simulink model "CoupledTanks"  (Simulink 6.5)
settings: Solver=ode45  StartTime=0.0  StopTime=2000  MaxStep=1e-1  RelTol=1e-3
InitFcn:
  | g = 9.81; %gravitational constant
  | 
  | % showVR = 1; %show VR world
  | % h1_init = 0; %initial condition
  | % h2_init = 0; %initial condition
libraries: vrlib x7
CloseFcn:
  | vrclose all;
  | clear figureVR worldVR;
settings Model: Creator=H  LastModifiedBy=Roubalj

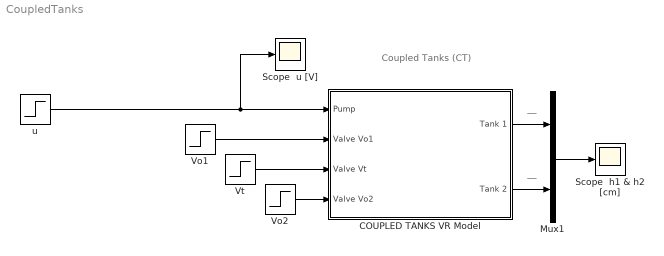
== system CoupledTanks ==
  note: Coupled Tanks (CT)
  note: __
  note: __
  COUPLED TANKS VR Model : Subsystem  mask(Coupled Tanks (CT) in laboratory K26){showVR=on, sfcnParam1=0, sfcnParam2=0}
      mask prompts: showVR "Show VirtualWorld?"; sfcnParam1 "Initial fluid level in the left tank 1   h1(0)  [cm]"; sfcnParam2 "Initial fluid  level in the right tank 2   h2 (0) [cm]"
      mask help:
      | Coupled Tanks (CT) in laboratory K26 - Virtual Reality
      | Real-Time Workshop generated S-function.
      mask Help:
      | Couple Tanks in laboratory K26 - Virtual Reality. <br><br>
      | 
      | 
      | This is a&nbsp;virtual model of the Coupled Tanks apparatus in Laboratory of automatic control
      | theory&nbsp;26 (<a href="http://support.dce.felk.cvut.cz/lab26/" target="_blank">http://support.dce.felk.cvut.cz/lab26/</a>),
      | which consists of a&nbsp;gear-pump, two tanks (left and right), inflow and outflow pipes and transfer (V<sub>t</sub>) and
      | output valves (V<sub>o1</sub>, V<sub>o2</sub>). The&nbsp;left tank is filled with the&nbsp;fluid by the&nbsp;gear-pump
      | controller by the&nbsp;voltage&nbsp;<em>u</em>&nbsp;[V]. The&nbsp;fluid can drain from the&nbsp;left tank through
      | the&nbsp;valve&nbsp;<em>v</em><sub>o1</sub>&nbsp;[%] or can drain to the&nbsp;right tank through the&nbsp;transfer
      | valve&nbsp;<em>v</em><sub>t</sub>&nbsp;[%]. The&nbsp;fluid drains away from the&nbsp;right tank through
      | the&nbsp;valve&nbsp;<em>v</em><sub>o2</sub>&nbsp;[%].<br><br>
      | 
      | The&nbsp;system input are the&nbsp;voltage of the&nbsp;motor of the&nbsp;gear-pump&nbsp;<em>u</em>&nbsp;[V]
      | and the&nbsp;opening of
      | the&nbsp;valves&nbsp;<em>v</em><sub>o1</sub>,&nbsp;<em>v</em><sub>t</sub>,&nbsp;<em>v</em><sub>o2</sub>&nbsp;[%].
      | The&nbsp;system outputs are the&nbsp;levels of the&nbsp;fluid in
      | the&nbsp;tanks&nbsp;<em>h</em><sub>1</sub>,&nbsp;<em>h</em><sub>2</sub>&nbsp;[cm].
      | The&nbsp;dynamics of the&nbsp;gear-pump is neglected. More information can be found on the&nbsp;website
      | <a href="http://support.dce.felk.cvut.cz/lab26/" target="_blank">http://support.dce.felk.cvut.cz/lab26/</a>.<br><br>
      | 
      | 
      | In the mask of the model, it can be set:
      | <ul>
      | <li>Initial fluid level in the left tank</li>
      | <li>Initial fluid level in the right tank.</li>
      | </ul><br><br>
      | 
      | 
      | Copyright: 2008, Jan Kricka, Jirka Roubal, Petr Husek.
      mask CallbackString:
      | if strcmp('off',get_param(gcb,'showVR'))
      |     vrclose all;
      | else
      |     if exist('figureVR')==0
      |         figureVR = vrfigure;
      |     end
      |     if exist('worldVR')==0
      |         worldVR = vrworld('CoupledTanks_VR.WRL');
      |     end
      | 	if isvalid(figureVR)==0
      |         open(worldVR);
      |         figureVR = vrfigure(worldVR,[650 80 550 350]);
      | 	end
      | end||
      mask Display:
      | image(imread('CoupledTanks_Image.jpg'));
      | port_label ('input',1,'u [V]');
      | port_label ('input',2,'Vo1 [-]');
      | port_label ('input',3,'Vt [-]');
      | port_label ('input',4,'Vo2 [-]');
      | port_label ('output',1,'h1 [cm]');
      | port_label ('output',2,'h2 [cm]');
  Mux1 : Mux  Inputs=2
  Scope  h1 & h2 [cm] : Scope
      settings: TimeRange=2000  YMin=0  YMax=30  SaveName=ty  DataFormat=Array  MaxDataPoints=500000
  Scope  u [V] : Scope
      settings: TimeRange=2000  YMin=0  YMax=12  SaveName=tu  DataFormat=Array  MaxDataPoints=500000
  Vo1 : Step  Time=0  After=0  SampleTime=0
  Vo2 : Step  Time=0  After=0.60  SampleTime=0
  Vt : Step  Time=0  SampleTime=0
  u : Step  Time=1000  Before=5  After=5*1.05  SampleTime=0
  wires:
  COUPLED TANKS VR Model/1(Tank 1) -> Mux1/1
  Mux1/1 -> Scope  h1 & h2 [cm]/1
  Vo1/1 -> COUPLED TANKS VR Model/2(Valve Vo1)
  Vt/1 -> COUPLED TANKS VR Model/3(Valve Vt)
  Vo2/1 -> COUPLED TANKS VR Model/4(Valve Vo2)
  u/1 -> Scope  u [V]/1, COUPLED TANKS VR Model/1(Pump)
  COUPLED TANKS VR Model/2(Tank 2) -> Mux1/2

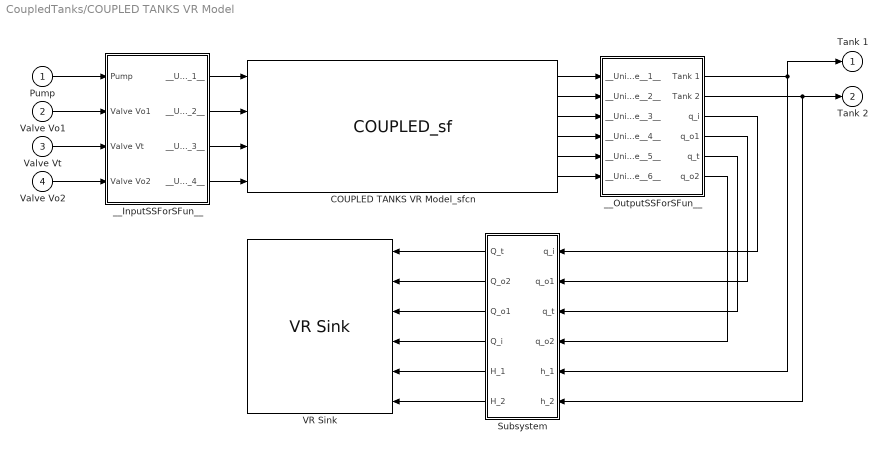
== system CoupledTanks/COUPLED TANKS VR Model ==
  Pump : Inport
  Valve Vo1 : Inport  Port=2
  Valve Vt : Inport  Port=3
  Valve Vo2 : Inport  Port=4
  COUPLED TANKS VR Model_sfcn : S-Function  FunctionName=COUPLED_sf  Parameters=sfcnParam1, sfcnParam2  SFunctionModules=""  mask{rtw_sf_name=COUPLED_sf, showVar=off, sfcnParam1=sfcnParam1, sfcnParam2=sfcnParam2}
      mask prompts: rtw_sf_name "Generated S-function name (model_sf):"; showVar "Show module list"; sfcnParam1 "h1_init:"; sfcnParam2 "h2_init:"
      mask help: Real-Time Workshop generated S-function.
      mask init:
      | displist = '';
      | if ~strcmp(get_param(gcb, 'FunctionName'), rtw_sf_name);
      |   set_param(gcb, 'FunctionName', rtw_sf_name);
      | end
      | % Check if we are generating RTW code
      | rtw_mode = false;
      | if strcmpi(get_param(bdroot(gcb),'SimulationStatus'),'Initializing')
      | 	rtw_mode = strcmpi(get_param(bdroot(gcb),'BuildingRTWCode'),'on') && ...
      | 		~strcmpi(get_param(bdroot(gcb),'TargetStyle'),'SimulationTarget');
      | end
      | if showVar || rtw_mode
      | 	if exist('rtwsfunc') == 2 | exist('rtwsfunc') == 6
      | 		tmplist = rtwsfunc(rtw_sf_name,gcb);
      | 		tmplist = ['\nList of Modules:\n', tmplist];
      | 	elseif showVar
      | 		tmplist = '\nList of Modules:\nRTW not licensed\n';
      |  	end
      | end
      | if showVar
      |   displist = tmplist;
      | end
      settings: CopyFcn=set_param(gcb,'LinkStatus','none');
      mask Help: helpview([docroot,'\toolbox\rtw\helptargets.map'],'rtw_Sfunc_target');
      mask Display:
      | port_label('input',1,'Pump');
      | port_label('input',2,'Valve Vo1');
      | port_label('input',3,'Valve Vt');
      | port_label('input',4,'Valve Vo2');
      | port_label('output',1,'Tank 1');
      | port_label('output',2,'Tank 2');
      | port_label('output',3,'q_i');
      | port_label('output',4,'q_o1');
      | port_label('output',5,'q_t');
      | port_label('output',6,'q_o2');
  Subsystem : Subsystem  Orientation=left
  VR Sink : vrlib/VR Sink  Orientation=left  SampleTime=-1  ViewEnable=on  RemoteChange=off  RemoteView=on  FieldsWritten=Valve_t.rotation.4.1.double#Valve_o2.rotation.4.1.double#Valve_o1.rotation.4.1.double#Pump.rotation.4.1.double#water1.scale.3.1.double#water2.scale.3.1.double  WorldFileName=CoupledTanks_VR.WRL  AutoView=off  FigureProperties={}
  __InputSSForSFun__ : Subsystem
  __OutputSSForSFun__ : Subsystem
  Tank 1 : Outport  PortDimensions=1  SampleTime=[-1 0]  DataType=double
  Tank 2 : Outport  Port=2  PortDimensions=1  SampleTime=[-1 0]  DataType=double
  wires:
  __OutputSSForSFun__/6(q_o2) -> Subsystem/4(q_o2)
  __OutputSSForSFun__/5(q_t) -> Subsystem/3(q_t)
  __OutputSSForSFun__/4(q_o1) -> Subsystem/2(q_o1)
  __OutputSSForSFun__/3(q_i) -> Subsystem/1(q_i)
  Subsystem/2(Q_o2) -> VR Sink/2
  Subsystem/3(Q_o1) -> VR Sink/3
  Subsystem/4(Q_i) -> VR Sink/4
  Subsystem/1(Q_t) -> VR Sink/1
  Subsystem/6(H_2) -> VR Sink/6
  Subsystem/5(H_1) -> VR Sink/5
  __OutputSSForSFun__/2(Tank 2) -> Subsystem/6(h_2), Tank 2/1
  __OutputSSForSFun__/1(Tank 1) -> Tank 1/1, Subsystem/5(h_1)
  COUPLED TANKS VR Model_sfcn/6 -> __OutputSSForSFun__/6(__UniqueInportName__6__)
  COUPLED TANKS VR Model_sfcn/5 -> __OutputSSForSFun__/5(__UniqueInportName__5__)
  COUPLED TANKS VR Model_sfcn/4 -> __OutputSSForSFun__/4(__UniqueInportName__4__)
  COUPLED TANKS VR Model_sfcn/3 -> __OutputSSForSFun__/3(__UniqueInportName__3__)
  COUPLED TANKS VR Model_sfcn/2 -> __OutputSSForSFun__/2(__UniqueInportName__2__)
  COUPLED TANKS VR Model_sfcn/1 -> __OutputSSForSFun__/1(__UniqueInportName__1__)
  __InputSSForSFun__/4(__UniqueOutportName__4__) -> COUPLED TANKS VR Model_sfcn/4
  __InputSSForSFun__/3(__UniqueOutportName__3__) -> COUPLED TANKS VR Model_sfcn/3
  __InputSSForSFun__/2(__UniqueOutportName__2__) -> COUPLED TANKS VR Model_sfcn/2
  __InputSSForSFun__/1(__UniqueOutportName__1__) -> COUPLED TANKS VR Model_sfcn/1
  Valve Vo2/1 -> __InputSSForSFun__/4(Valve Vo2)
  Valve Vt/1 -> __InputSSForSFun__/3(Valve Vt)
  Valve Vo1/1 -> __InputSSForSFun__/2(Valve Vo1)
  Pump/1 -> __InputSSForSFun__/1(Pump)

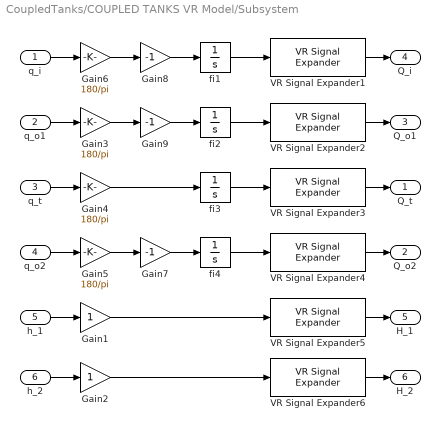
== system CoupledTanks/COUPLED TANKS VR Model/Subsystem ==
  q_i : Inport
  q_o1 : Inport  Port=2
  q_t : Inport  Port=3
  q_o2 : Inport  Port=4
  h_1 : Inport  Port=5
  h_2 : Inport  Port=6
  Gain1 : Gain
  Gain2 : Gain
  Gain{3..6} (4 alike) : Gain  Gain=180/pi
  Gain7 : Gain  Gain=-1
  Gain8 : Gain  Gain=-1
  Gain9 : Gain  Gain=-1
  VR Signal Expander{1..4} (4 alike) : vrlib/VR Signal Expander  SystemSampleTime=-1  outwidth=4  outidx=[4]
  VR Signal Expander5 : vrlib/VR Signal Expander  SystemSampleTime=-1  outwidth=3  outidx=[2]
  VR Signal Expander6 : vrlib/VR Signal Expander  SystemSampleTime=-1  outwidth=3  outidx=[2]
  fi{1..4} (4 alike) : Integrator
  Q_t : Outport
  Q_o2 : Outport  Port=2
  Q_o1 : Outport  Port=3
  Q_i : Outport  Port=4
  H_1 : Outport  Port=5
  H_2 : Outport  Port=6
  wires:
  Gain9/1 -> fi2/1
  Gain8/1 -> fi1/1
  Gain7/1 -> fi4/1
  Gain5/1 -> Gain7/1
  q_o2/1 -> Gain5/1
  VR Signal Expander4/1 -> Q_o2/1
  fi4/1 -> VR Signal Expander4/1
  Gain4/1 -> fi3/1
  Gain6/1 -> Gain8/1
  Gain3/1 -> Gain9/1
  q_t/1 -> Gain4/1
  q_o1/1 -> Gain3/1
  Gain2/1 -> VR Signal Expander6/1
  Gain1/1 -> VR Signal Expander5/1
  VR Signal Expander6/1 -> H_2/1
  VR Signal Expander5/1 -> H_1/1
  VR Signal Expander1/1 -> Q_i/1
  VR Signal Expander2/1 -> Q_o1/1
  VR Signal Expander3/1 -> Q_t/1
  h_2/1 -> Gain2/1
  h_1/1 -> Gain1/1
  q_i/1 -> Gain6/1
  fi2/1 -> VR Signal Expander2/1
  fi3/1 -> VR Signal Expander3/1
  fi1/1 -> VR Signal Expander1/1

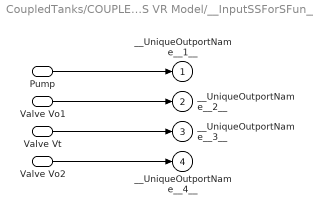
== system CoupledTanks/COUPLED TANKS VR Model/__InputSSForSFun__ ==
  Pump : Inport
  Valve Vo1 : Inport  Port=2
  Valve Vt : Inport  Port=3
  Valve Vo2 : Inport  Port=4
  __UniqueOutportName__1__ : Outport
  __UniqueOutportName__2__ : Outport  Port=2
  __UniqueOutportName__3__ : Outport  Port=3
  __UniqueOutportName__4__ : Outport  Port=4
  wires:
  Valve Vo2/1 -> __UniqueOutportName__4__/1
  Valve Vt/1 -> __UniqueOutportName__3__/1
  Valve Vo1/1 -> __UniqueOutportName__2__/1
  Pump/1 -> __UniqueOutportName__1__/1

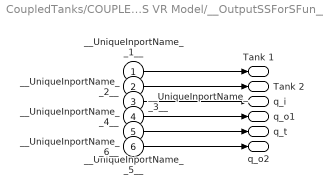
== system CoupledTanks/COUPLED TANKS VR Model/__OutputSSForSFun__ ==
  __UniqueInportName__1__ : Inport
  __UniqueInportName__2__ : Inport  Port=2
  __UniqueInportName__3__ : Inport  Port=3
  __UniqueInportName__4__ : Inport  Port=4
  __UniqueInportName__5__ : Inport  Port=5
  __UniqueInportName__6__ : Inport  Port=6
  Tank 1 : Outport  PortDimensions=1  SampleTime=[-1 0]  DataType=double
  Tank 2 : Outport  Port=2  PortDimensions=1  SampleTime=[-1 0]  DataType=double
  q_i : Outport  Port=3  PortDimensions=1  SampleTime=[0 1]  DataType=double
  q_o1 : Outport  Port=4  PortDimensions=1  SampleTime=[-1 0]  DataType=double
  q_t : Outport  Port=5  PortDimensions=1  SampleTime=[-1 0]  DataType=double
  q_o2 : Outport  Port=6  PortDimensions=1  SampleTime=[-1 0]  DataType=double
  wires:
  __UniqueInportName__6__/1 -> q_o2/1
  __UniqueInportName__5__/1 -> q_t/1
  __UniqueInportName__4__/1 -> q_o1/1
  __UniqueInportName__3__/1 -> q_i/1
  __UniqueInportName__2__/1 -> Tank 2/1
  __UniqueInportName__1__/1 -> Tank 1/1
